simulink model "AariaHIABTorqueR2017a2"  (R2017a)
settings: Solver=VariableStepAuto  StartTime=0.0  StopTime=inf  FixedStep=0.1  RelTol=1e-3  EnableMultiTasking=on
model workspace (MATLAB code in the model file):
  | my_a =1;
undefined symbols (not defined in the file or in its folder): AARIAENV, AARIAMAN, AARIASEN, Camera, sensor, Source_TS, X, Y, Z
libraries: sm_lib x369, nesl_utility x225, dspmathops x92, simulink x70, powerlib_meascontrol x3, vrlib x2, aerolibanimutils x1, aerolibutil x1
(part 9 of 10)

== system AariaHIABTorqueR2017a2/Joint2/RevoluteMotion/IMU Sensors/Sensor Module1/omega_noise ==
  Cumulative Sum : dspmathops/Cumulative Sum  dim=Channels (running sum)  InputProcessing=Columns as channels (frame based)  reset_popup=None  outputDataTypeStr=Inherit: Same as accumulator  outputLastDataTypeStr=Inherit: Same as accumulator  outputMin=[]  outputMax=[]  roundingMode=Floor  overflowMode=off
      settings: SourceProductName=DSP System Toolbox
  Cumulative Sum1 : dspmathops/Cumulative Sum  dim=Channels (running sum)  InputProcessing=Columns as channels (frame based)  reset_popup=None  outputDataTypeStr=Inherit: Same as accumulator  outputLastDataTypeStr=Inherit: Same as accumulator  outputMin=[]  outputMax=[]  roundingMode=Floor  overflowMode=off
      settings: SourceProductName=DSP System Toolbox
  Cumulative Sum2 : dspmathops/Cumulative Sum  dim=Channels (running sum)  InputProcessing=Columns as channels (frame based)  reset_popup=None  outputDataTypeStr=Inherit: Same as accumulator  outputLastDataTypeStr=Inherit: Same as accumulator  outputMin=[]  outputMax=[]  roundingMode=Floor  overflowMode=off
      settings: SourceProductName=DSP System Toolbox
  Gain1 : Gain  Gain=AARIASEN.ErrorGain
  Gain2 : Gain  Gain=AARIASEN.gNormalGain
  Gain3 : Gain  Gain=AARIASEN.gNormalGain
  Gain4 : Gain  Gain=AARIASEN.gNormalGain
  Mux5 : Mux  Inputs=3
  Random Number : RandomNumber  Mean=AARIASEN.gMu  Variance=AARIASEN.gSigma  Seed=AARIASEN.rand(nL,(nS-1)*6+1)  SampleTime=AARIAENV.Source_TS
  Random Number1 : RandomNumber  Mean=AARIASEN.gMu  Variance=AARIASEN.gSigma  Seed=AARIASEN.rand(nL,(nS-1)*6+2)  SampleTime=AARIAENV.Source_TS
  Random Number2 : RandomNumber  Mean=AARIASEN.gMu  Variance=AARIASEN.gSigma  Seed=AARIASEN.rand(nL,(nS-1)*6+3)  SampleTime=AARIAENV.Source_TS
  Sum1 : Sum  Inputs=|++
  Sum2 : Sum  Inputs=|++
  Sum3 : Sum  Inputs=++|
  Sum4 : Sum  Inputs=|++
  gyro in-run bias : simulink/Sources/Ramp  slope=AARIASEN.gBias  start=0  X0=AARIASEN.gInitBias
  gyro random walk : UniformRandomNumber  Minimum=-AARIASEN.gWalk  Maximum=AARIASEN.gWalk  Seed=AARIASEN.rand(nL,(nS-1)*6+1)  SampleTime=AARIAENV.Source_TS
  gyro random walk1 : UniformRandomNumber  Minimum=-AARIASEN.gWalk  Maximum=AARIASEN.gWalk  Seed=AARIASEN.rand(nL,(nS-1)*6+2)  SampleTime=AARIAENV.Source_TS
  gyro random walk2 : UniformRandomNumber  Minimum=-AARIASEN.gWalk  Maximum=AARIASEN.gWalk  Seed=AARIASEN.rand(nL,(nS-1)*6+3)  SampleTime=AARIAENV.Source_TS
  noise : Outport
  wires:
  Gain4/1 -> Sum4/1
  Gain3/1 -> Sum2/1
  Gain2/1 -> Sum1/1
  Random Number/1 -> Gain2/1
  Random Number1/1 -> Gain3/1
  Random Number2/1 -> Gain4/1
  Sum3/1 -> Gain1/1
  Mux5/1 -> Sum3/2
  Sum4/1 -> Mux5/3
  Cumulative Sum2/1 -> Sum4/2
  Cumulative Sum1/1 -> Sum2/2
  Sum2/1 -> Mux5/2
  Sum1/1 -> Mux5/1
  gyro random walk2/1 -> Cumulative Sum2/1
  gyro random walk1/1 -> Cumulative Sum1/1
  Gain1/1 -> noise/1
  gyro random walk/1 -> Cumulative Sum/1
  Cumulative Sum/1 -> Sum1/2
  gyro in-run bias/1 -> Sum3/1

== system AariaHIABTorqueR2017a2/Joint2/RevoluteMotion/IMU Sensors/Sensor Module2/a_noise ==
  Cumulative Sum1 : dspmathops/Cumulative Sum  dim=Channels (running sum)  InputProcessing=Columns as channels (frame based)  reset_popup=None  outputDataTypeStr=Inherit: Same as accumulator  outputLastDataTypeStr=Inherit: Same as accumulator  outputMin=[]  outputMax=[]  roundingMode=Floor  overflowMode=off
      settings: SourceProductName=DSP System Toolbox
  Cumulative Sum2 : dspmathops/Cumulative Sum  dim=Channels (running sum)  InputProcessing=Columns as channels (frame based)  reset_popup=None  outputDataTypeStr=Inherit: Same as accumulator  outputLastDataTypeStr=Inherit: Same as accumulator  outputMin=[]  outputMax=[]  roundingMode=Floor  overflowMode=off
      settings: SourceProductName=DSP System Toolbox
  Cumulative Sum3 : dspmathops/Cumulative Sum  dim=Channels (running sum)  InputProcessing=Columns as channels (frame based)  reset_popup=None  outputDataTypeStr=Inherit: Same as accumulator  outputLastDataTypeStr=Inherit: Same as accumulator  outputMin=[]  outputMax=[]  roundingMode=Floor  overflowMode=off
      settings: SourceProductName=DSP System Toolbox
  Gain1 : Gain  Gain=9.81
  Gain2 : Gain  Gain=AARIASEN.ErrorGain
  Gain3 : Gain  Gain=9.81
  Gain4 : Gain  Gain=AARIASEN.aNormalGain
  Gain5 : Gain  Gain=9.81
  Gain6 : Gain  Gain=AARIASEN.aNormalGain
  Gain7 : Gain  Gain=AARIASEN.aNormalGain
  Mux5 : Mux  Inputs=3
  Random Number : RandomNumber  Mean=AARIASEN.aMu  Variance=AARIASEN.aSigma  Seed=AARIASEN.rand(nL,(nS-1)*6+4)  SampleTime=AARIAENV.Source_TS
  Random Number1 : RandomNumber  Mean=AARIASEN.aMu  Variance=AARIASEN.aSigma  Seed=AARIASEN.rand(nL,(nS-1)*6+5)  SampleTime=AARIAENV.Source_TS
  Random Number2 : RandomNumber  Mean=AARIASEN.aMu  Variance=AARIASEN.aSigma  Seed=AARIASEN.rand(nL,(nS-1)*6+6)  SampleTime=AARIAENV.Source_TS
  Sum1 : Sum  Inputs=|++
  Sum2 : Sum  Inputs=|++
  Sum3 : Sum  Inputs=|++
  Sum4 : Sum  Inputs=++|
  acc in-run bias : simulink/Sources/Ramp  slope=AARIASEN.aBias  start=0  X0=AARIASEN.aInitBias
  acc random walk : UniformRandomNumber  Minimum=-AARIASEN.aWalk  Maximum=AARIASEN.aWalk  Seed=AARIASEN.rand(nL,(nS-1)*6+4)  SampleTime=AARIAENV.Source_TS
  acc random walk1 : UniformRandomNumber  Minimum=-AARIASEN.aWalk  Maximum=AARIASEN.aWalk  Seed=AARIASEN.rand(nL,(nS-1)*6+5)  SampleTime=AARIAENV.Source_TS
  acc random walk2 : UniformRandomNumber  Minimum=-AARIASEN.aWalk  Maximum=AARIASEN.aWalk  Seed=AARIASEN.rand(nL,(nS-1)*6+6)  SampleTime=AARIAENV.Source_TS
  noise : Outport
  wires:
  Gain7/1 -> Gain3/1
  Gain6/1 -> Gain5/1
  Gain4/1 -> Gain1/1
  Random Number2/1 -> Gain7/1
  Random Number1/1 -> Gain6/1
  Random Number/1 -> Gain4/1
  Gain3/1 -> Sum3/1
  Gain5/1 -> Sum2/1
  Gain1/1 -> Sum1/1
  Sum4/1 -> Gain2/1
  Mux5/1 -> Sum4/2
  acc random walk2/1 -> Cumulative Sum3/1
  acc random walk1/1 -> Cumulative Sum1/1
  Sum2/1 -> Mux5/2
  Cumulative Sum1/1 -> Sum2/2
  Sum3/1 -> Mux5/3
  Sum1/1 -> Mux5/1
  Cumulative Sum2/1 -> Sum1/2
  Cumulative Sum3/1 -> Sum3/2
  Gain2/1 -> noise/1
  acc in-run bias/1 -> Sum4/1
  acc random walk/1 -> Cumulative Sum2/1

== system AariaHIABTorqueR2017a2/Joint2/RevoluteMotion/IMU Sensors/Sensor Module2/omega_noise ==
  Cumulative Sum : dspmathops/Cumulative Sum  dim=Channels (running sum)  InputProcessing=Columns as channels (frame based)  reset_popup=None  outputDataTypeStr=Inherit: Same as accumulator  outputLastDataTypeStr=Inherit: Same as accumulator  outputMin=[]  outputMax=[]  roundingMode=Floor  overflowMode=off
      settings: SourceProductName=DSP System Toolbox
  Cumulative Sum1 : dspmathops/Cumulative Sum  dim=Channels (running sum)  InputProcessing=Columns as channels (frame based)  reset_popup=None  outputDataTypeStr=Inherit: Same as accumulator  outputLastDataTypeStr=Inherit: Same as accumulator  outputMin=[]  outputMax=[]  roundingMode=Floor  overflowMode=off
      settings: SourceProductName=DSP System Toolbox
  Cumulative Sum2 : dspmathops/Cumulative Sum  dim=Channels (running sum)  InputProcessing=Columns as channels (frame based)  reset_popup=None  outputDataTypeStr=Inherit: Same as accumulator  outputLastDataTypeStr=Inherit: Same as accumulator  outputMin=[]  outputMax=[]  roundingMode=Floor  overflowMode=off
      settings: SourceProductName=DSP System Toolbox
  Gain1 : Gain  Gain=AARIASEN.ErrorGain
  Gain2 : Gain  Gain=AARIASEN.gNormalGain
  Gain3 : Gain  Gain=AARIASEN.gNormalGain
  Gain4 : Gain  Gain=AARIASEN.gNormalGain
  Mux5 : Mux  Inputs=3
  Random Number : RandomNumber  Mean=AARIASEN.gMu  Variance=AARIASEN.gSigma  Seed=AARIASEN.rand(nL,(nS-1)*6+1)  SampleTime=AARIAENV.Source_TS
  Random Number1 : RandomNumber  Mean=AARIASEN.gMu  Variance=AARIASEN.gSigma  Seed=AARIASEN.rand(nL,(nS-1)*6+2)  SampleTime=AARIAENV.Source_TS
  Random Number2 : RandomNumber  Mean=AARIASEN.gMu  Variance=AARIASEN.gSigma  Seed=AARIASEN.rand(nL,(nS-1)*6+3)  SampleTime=AARIAENV.Source_TS
  Sum1 : Sum  Inputs=|++
  Sum2 : Sum  Inputs=|++
  Sum3 : Sum  Inputs=++|
  Sum4 : Sum  Inputs=|++
  gyro in-run bias : simulink/Sources/Ramp  slope=AARIASEN.gBias  start=0  X0=AARIASEN.gInitBias
  gyro random walk : UniformRandomNumber  Minimum=-AARIASEN.gWalk  Maximum=AARIASEN.gWalk  Seed=AARIASEN.rand(nL,(nS-1)*6+1)  SampleTime=AARIAENV.Source_TS
  gyro random walk1 : UniformRandomNumber  Minimum=-AARIASEN.gWalk  Maximum=AARIASEN.gWalk  Seed=AARIASEN.rand(nL,(nS-1)*6+2)  SampleTime=AARIAENV.Source_TS
  gyro random walk2 : UniformRandomNumber  Minimum=-AARIASEN.gWalk  Maximum=AARIASEN.gWalk  Seed=AARIASEN.rand(nL,(nS-1)*6+3)  SampleTime=AARIAENV.Source_TS
  noise : Outport
  wires:
  Gain4/1 -> Sum4/1
  Gain3/1 -> Sum2/1
  Gain2/1 -> Sum1/1
  Random Number/1 -> Gain2/1
  Random Number1/1 -> Gain3/1
  Random Number2/1 -> Gain4/1
  Sum3/1 -> Gain1/1
  Mux5/1 -> Sum3/2
  Sum4/1 -> Mux5/3
  Cumulative Sum2/1 -> Sum4/2
  Cumulative Sum1/1 -> Sum2/2
  Sum2/1 -> Mux5/2
  Sum1/1 -> Mux5/1
  gyro random walk2/1 -> Cumulative Sum2/1
  gyro random walk1/1 -> Cumulative Sum1/1
  Gain1/1 -> noise/1
  gyro random walk/1 -> Cumulative Sum/1
  Cumulative Sum/1 -> Sum1/2
  gyro in-run bias/1 -> Sum3/1

== system AariaHIABTorqueR2017a2/Joint3/RevoluteMotion/IMU Sensors/Sensor Module1/a_noise ==
  Cumulative Sum1 : dspmathops/Cumulative Sum  dim=Channels (running sum)  InputProcessing=Columns as channels (frame based)  reset_popup=None  outputDataTypeStr=Inherit: Same as accumulator  outputLastDataTypeStr=Inherit: Same as accumulator  outputMin=[]  outputMax=[]  roundingMode=Floor  overflowMode=off
      settings: SourceProductName=DSP System Toolbox
  Cumulative Sum2 : dspmathops/Cumulative Sum  dim=Channels (running sum)  InputProcessing=Columns as channels (frame based)  reset_popup=None  outputDataTypeStr=Inherit: Same as accumulator  outputLastDataTypeStr=Inherit: Same as accumulator  outputMin=[]  outputMax=[]  roundingMode=Floor  overflowMode=off
      settings: SourceProductName=DSP System Toolbox
  Cumulative Sum3 : dspmathops/Cumulative Sum  dim=Channels (running sum)  InputProcessing=Columns as channels (frame based)  reset_popup=None  outputDataTypeStr=Inherit: Same as accumulator  outputLastDataTypeStr=Inherit: Same as accumulator  outputMin=[]  outputMax=[]  roundingMode=Floor  overflowMode=off
      settings: SourceProductName=DSP System Toolbox
  Gain1 : Gain  Gain=9.81
  Gain2 : Gain  Gain=AARIASEN.ErrorGain
  Gain3 : Gain  Gain=9.81
  Gain4 : Gain  Gain=AARIASEN.aNormalGain
  Gain5 : Gain  Gain=9.81
  Gain6 : Gain  Gain=AARIASEN.aNormalGain
  Gain7 : Gain  Gain=AARIASEN.aNormalGain
  Mux5 : Mux  Inputs=3
  Random Number : RandomNumber  Mean=AARIASEN.aMu  Variance=AARIASEN.aSigma  Seed=AARIASEN.rand(nL,(nS-1)*6+4)  SampleTime=AARIAENV.Source_TS
  Random Number1 : RandomNumber  Mean=AARIASEN.aMu  Variance=AARIASEN.aSigma  Seed=AARIASEN.rand(nL,(nS-1)*6+5)  SampleTime=AARIAENV.Source_TS
  Random Number2 : RandomNumber  Mean=AARIASEN.aMu  Variance=AARIASEN.aSigma  Seed=AARIASEN.rand(nL,(nS-1)*6+6)  SampleTime=AARIAENV.Source_TS
  Sum1 : Sum  Inputs=|++
  Sum2 : Sum  Inputs=|++
  Sum3 : Sum  Inputs=|++
  Sum4 : Sum  Inputs=++|
  acc in-run bias : simulink/Sources/Ramp  slope=AARIASEN.aBias  start=0  X0=AARIASEN.aInitBias
  acc random walk : UniformRandomNumber  Minimum=-AARIASEN.aWalk  Maximum=AARIASEN.aWalk  Seed=AARIASEN.rand(nL,(nS-1)*6+4)  SampleTime=AARIAENV.Source_TS
  acc random walk1 : UniformRandomNumber  Minimum=-AARIASEN.aWalk  Maximum=AARIASEN.aWalk  Seed=AARIASEN.rand(nL,(nS-1)*6+5)  SampleTime=AARIAENV.Source_TS
  acc random walk2 : UniformRandomNumber  Minimum=-AARIASEN.aWalk  Maximum=AARIASEN.aWalk  Seed=AARIASEN.rand(nL,(nS-1)*6+6)  SampleTime=AARIAENV.Source_TS
  noise : Outport
  wires:
  Gain7/1 -> Gain3/1
  Gain6/1 -> Gain5/1
  Gain4/1 -> Gain1/1
  Random Number2/1 -> Gain7/1
  Random Number1/1 -> Gain6/1
  Random Number/1 -> Gain4/1
  Gain3/1 -> Sum3/1
  Gain5/1 -> Sum2/1
  Gain1/1 -> Sum1/1
  Sum4/1 -> Gain2/1
  Mux5/1 -> Sum4/2
  acc random walk2/1 -> Cumulative Sum3/1
  acc random walk1/1 -> Cumulative Sum1/1
  Sum2/1 -> Mux5/2
  Cumulative Sum1/1 -> Sum2/2
  Sum3/1 -> Mux5/3
  Sum1/1 -> Mux5/1
  Cumulative Sum2/1 -> Sum1/2
  Cumulative Sum3/1 -> Sum3/2
  Gain2/1 -> noise/1
  acc in-run bias/1 -> Sum4/1
  acc random walk/1 -> Cumulative Sum2/1

== system AariaHIABTorqueR2017a2/Joint3/RevoluteMotion/IMU Sensors/Sensor Module1/omega_noise ==
  Cumulative Sum : dspmathops/Cumulative Sum  dim=Channels (running sum)  InputProcessing=Columns as channels (frame based)  reset_popup=None  outputDataTypeStr=Inherit: Same as accumulator  outputLastDataTypeStr=Inherit: Same as accumulator  outputMin=[]  outputMax=[]  roundingMode=Floor  overflowMode=off
      settings: SourceProductName=DSP System Toolbox
  Cumulative Sum1 : dspmathops/Cumulative Sum  dim=Channels (running sum)  InputProcessing=Columns as channels (frame based)  reset_popup=None  outputDataTypeStr=Inherit: Same as accumulator  outputLastDataTypeStr=Inherit: Same as accumulator  outputMin=[]  outputMax=[]  roundingMode=Floor  overflowMode=off
      settings: SourceProductName=DSP System Toolbox
  Cumulative Sum2 : dspmathops/Cumulative Sum  dim=Channels (running sum)  InputProcessing=Columns as channels (frame based)  reset_popup=None  outputDataTypeStr=Inherit: Same as accumulator  outputLastDataTypeStr=Inherit: Same as accumulator  outputMin=[]  outputMax=[]  roundingMode=Floor  overflowMode=off
      settings: SourceProductName=DSP System Toolbox
  Gain1 : Gain  Gain=AARIASEN.ErrorGain
  Gain2 : Gain  Gain=AARIASEN.gNormalGain
  Gain3 : Gain  Gain=AARIASEN.gNormalGain
  Gain4 : Gain  Gain=AARIASEN.gNormalGain
  Mux5 : Mux  Inputs=3
  Random Number : RandomNumber  Mean=AARIASEN.gMu  Variance=AARIASEN.gSigma  Seed=AARIASEN.rand(nL,(nS-1)*6+1)  SampleTime=AARIAENV.Source_TS
  Random Number1 : RandomNumber  Mean=AARIASEN.gMu  Variance=AARIASEN.gSigma  Seed=AARIASEN.rand(nL,(nS-1)*6+2)  SampleTime=AARIAENV.Source_TS
  Random Number2 : RandomNumber  Mean=AARIASEN.gMu  Variance=AARIASEN.gSigma  Seed=AARIASEN.rand(nL,(nS-1)*6+3)  SampleTime=AARIAENV.Source_TS
  Sum1 : Sum  Inputs=|++
  Sum2 : Sum  Inputs=|++
  Sum3 : Sum  Inputs=++|
  Sum4 : Sum  Inputs=|++
  gyro in-run bias : simulink/Sources/Ramp  slope=AARIASEN.gBias  start=0  X0=AARIASEN.gInitBias
  gyro random walk : UniformRandomNumber  Minimum=-AARIASEN.gWalk  Maximum=AARIASEN.gWalk  Seed=AARIASEN.rand(nL,(nS-1)*6+1)  SampleTime=AARIAENV.Source_TS
  gyro random walk1 : UniformRandomNumber  Minimum=-AARIASEN.gWalk  Maximum=AARIASEN.gWalk  Seed=AARIASEN.rand(nL,(nS-1)*6+2)  SampleTime=AARIAENV.Source_TS
  gyro random walk2 : UniformRandomNumber  Minimum=-AARIASEN.gWalk  Maximum=AARIASEN.gWalk  Seed=AARIASEN.rand(nL,(nS-1)*6+3)  SampleTime=AARIAENV.Source_TS
  noise : Outport
  wires:
  Gain4/1 -> Sum4/1
  Gain3/1 -> Sum2/1
  Gain2/1 -> Sum1/1
  Random Number/1 -> Gain2/1
  Random Number1/1 -> Gain3/1
  Random Number2/1 -> Gain4/1
  Sum3/1 -> Gain1/1
  Mux5/1 -> Sum3/2
  Sum4/1 -> Mux5/3
  Cumulative Sum2/1 -> Sum4/2
  Cumulative Sum1/1 -> Sum2/2
  Sum2/1 -> Mux5/2
  Sum1/1 -> Mux5/1
  gyro random walk2/1 -> Cumulative Sum2/1
  gyro random walk1/1 -> Cumulative Sum1/1
  Gain1/1 -> noise/1
  gyro random walk/1 -> Cumulative Sum/1
  Cumulative Sum/1 -> Sum1/2
  gyro in-run bias/1 -> Sum3/1

== system AariaHIABTorqueR2017a2/Joint3/RevoluteMotion/IMU Sensors/Sensor Module2/a_noise ==
  Cumulative Sum1 : dspmathops/Cumulative Sum  dim=Channels (running sum)  InputProcessing=Columns as channels (frame based)  reset_popup=None  outputDataTypeStr=Inherit: Same as accumulator  outputLastDataTypeStr=Inherit: Same as accumulator  outputMin=[]  outputMax=[]  roundingMode=Floor  overflowMode=off
      settings: SourceProductName=DSP System Toolbox
  Cumulative Sum2 : dspmathops/Cumulative Sum  dim=Channels (running sum)  InputProcessing=Columns as channels (frame based)  reset_popup=None  outputDataTypeStr=Inherit: Same as accumulator  outputLastDataTypeStr=Inherit: Same as accumulator  outputMin=[]  outputMax=[]  roundingMode=Floor  overflowMode=off
      settings: SourceProductName=DSP System Toolbox
  Cumulative Sum3 : dspmathops/Cumulative Sum  dim=Channels (running sum)  InputProcessing=Columns as channels (frame based)  reset_popup=None  outputDataTypeStr=Inherit: Same as accumulator  outputLastDataTypeStr=Inherit: Same as accumulator  outputMin=[]  outputMax=[]  roundingMode=Floor  overflowMode=off
      settings: SourceProductName=DSP System Toolbox
  Gain1 : Gain  Gain=9.81
  Gain2 : Gain  Gain=AARIASEN.ErrorGain
  Gain3 : Gain  Gain=9.81
  Gain4 : Gain  Gain=AARIASEN.aNormalGain
  Gain5 : Gain  Gain=9.81
  Gain6 : Gain  Gain=AARIASEN.aNormalGain
  Gain7 : Gain  Gain=AARIASEN.aNormalGain
  Mux5 : Mux  Inputs=3
  Random Number : RandomNumber  Mean=AARIASEN.aMu  Variance=AARIASEN.aSigma  Seed=AARIASEN.rand(nL,(nS-1)*6+4)  SampleTime=AARIAENV.Source_TS
  Random Number1 : RandomNumber  Mean=AARIASEN.aMu  Variance=AARIASEN.aSigma  Seed=AARIASEN.rand(nL,(nS-1)*6+5)  SampleTime=AARIAENV.Source_TS
  Random Number2 : RandomNumber  Mean=AARIASEN.aMu  Variance=AARIASEN.aSigma  Seed=AARIASEN.rand(nL,(nS-1)*6+6)  SampleTime=AARIAENV.Source_TS
  Sum1 : Sum  Inputs=|++
  Sum2 : Sum  Inputs=|++
  Sum3 : Sum  Inputs=|++
  Sum4 : Sum  Inputs=++|
  acc in-run bias : simulink/Sources/Ramp  slope=AARIASEN.aBias  start=0  X0=AARIASEN.aInitBias
  acc random walk : UniformRandomNumber  Minimum=-AARIASEN.aWalk  Maximum=AARIASEN.aWalk  Seed=AARIASEN.rand(nL,(nS-1)*6+4)  SampleTime=AARIAENV.Source_TS
  acc random walk1 : UniformRandomNumber  Minimum=-AARIASEN.aWalk  Maximum=AARIASEN.aWalk  Seed=AARIASEN.rand(nL,(nS-1)*6+5)  SampleTime=AARIAENV.Source_TS
  acc random walk2 : UniformRandomNumber  Minimum=-AARIASEN.aWalk  Maximum=AARIASEN.aWalk  Seed=AARIASEN.rand(nL,(nS-1)*6+6)  SampleTime=AARIAENV.Source_TS
  noise : Outport
  wires:
  Gain7/1 -> Gain3/1
  Gain6/1 -> Gain5/1
  Gain4/1 -> Gain1/1
  Random Number2/1 -> Gain7/1
  Random Number1/1 -> Gain6/1
  Random Number/1 -> Gain4/1
  Gain3/1 -> Sum3/1
  Gain5/1 -> Sum2/1
  Gain1/1 -> Sum1/1
  Sum4/1 -> Gain2/1
  Mux5/1 -> Sum4/2
  acc random walk2/1 -> Cumulative Sum3/1
  acc random walk1/1 -> Cumulative Sum1/1
  Sum2/1 -> Mux5/2
  Cumulative Sum1/1 -> Sum2/2
  Sum3/1 -> Mux5/3
  Sum1/1 -> Mux5/1
  Cumulative Sum2/1 -> Sum1/2
  Cumulative Sum3/1 -> Sum3/2
  Gain2/1 -> noise/1
  acc in-run bias/1 -> Sum4/1
  acc random walk/1 -> Cumulative Sum2/1

== system AariaHIABTorqueR2017a2/Joint3/RevoluteMotion/IMU Sensors/Sensor Module2/omega_noise ==
  Cumulative Sum : dspmathops/Cumulative Sum  dim=Channels (running sum)  InputProcessing=Columns as channels (frame based)  reset_popup=None  outputDataTypeStr=Inherit: Same as accumulator  outputLastDataTypeStr=Inherit: Same as accumulator  outputMin=[]  outputMax=[]  roundingMode=Floor  overflowMode=off
      settings: SourceProductName=DSP System Toolbox
  Cumulative Sum1 : dspmathops/Cumulative Sum  dim=Channels (running sum)  InputProcessing=Columns as channels (frame based)  reset_popup=None  outputDataTypeStr=Inherit: Same as accumulator  outputLastDataTypeStr=Inherit: Same as accumulator  outputMin=[]  outputMax=[]  roundingMode=Floor  overflowMode=off
      settings: SourceProductName=DSP System Toolbox
  Cumulative Sum2 : dspmathops/Cumulative Sum  dim=Channels (running sum)  InputProcessing=Columns as channels (frame based)  reset_popup=None  outputDataTypeStr=Inherit: Same as accumulator  outputLastDataTypeStr=Inherit: Same as accumulator  outputMin=[]  outputMax=[]  roundingMode=Floor  overflowMode=off
      settings: SourceProductName=DSP System Toolbox
  Gain1 : Gain  Gain=AARIASEN.ErrorGain
  Gain2 : Gain  Gain=AARIASEN.gNormalGain
  Gain3 : Gain  Gain=AARIASEN.gNormalGain
  Gain4 : Gain  Gain=AARIASEN.gNormalGain
  Mux5 : Mux  Inputs=3
  Random Number : RandomNumber  Mean=AARIASEN.gMu  Variance=AARIASEN.gSigma  Seed=AARIASEN.rand(nL,(nS-1)*6+1)  SampleTime=AARIAENV.Source_TS
  Random Number1 : RandomNumber  Mean=AARIASEN.gMu  Variance=AARIASEN.gSigma  Seed=AARIASEN.rand(nL,(nS-1)*6+2)  SampleTime=AARIAENV.Source_TS
  Random Number2 : RandomNumber  Mean=AARIASEN.gMu  Variance=AARIASEN.gSigma  Seed=AARIASEN.rand(nL,(nS-1)*6+3)  SampleTime=AARIAENV.Source_TS
  Sum1 : Sum  Inputs=|++
  Sum2 : Sum  Inputs=|++
  Sum3 : Sum  Inputs=++|
  Sum4 : Sum  Inputs=|++
  gyro in-run bias : simulink/Sources/Ramp  slope=AARIASEN.gBias  start=0  X0=AARIASEN.gInitBias
  gyro random walk : UniformRandomNumber  Minimum=-AARIASEN.gWalk  Maximum=AARIASEN.gWalk  Seed=AARIASEN.rand(nL,(nS-1)*6+1)  SampleTime=AARIAENV.Source_TS
  gyro random walk1 : UniformRandomNumber  Minimum=-AARIASEN.gWalk  Maximum=AARIASEN.gWalk  Seed=AARIASEN.rand(nL,(nS-1)*6+2)  SampleTime=AARIAENV.Source_TS
  gyro random walk2 : UniformRandomNumber  Minimum=-AARIASEN.gWalk  Maximum=AARIASEN.gWalk  Seed=AARIASEN.rand(nL,(nS-1)*6+3)  SampleTime=AARIAENV.Source_TS
  noise : Outport
  wires:
  Gain4/1 -> Sum4/1
  Gain3/1 -> Sum2/1
  Gain2/1 -> Sum1/1
  Random Number/1 -> Gain2/1
  Random Number1/1 -> Gain3/1
  Random Number2/1 -> Gain4/1
  Sum3/1 -> Gain1/1
  Mux5/1 -> Sum3/2
  Sum4/1 -> Mux5/3
  Cumulative Sum2/1 -> Sum4/2
  Cumulative Sum1/1 -> Sum2/2
  Sum2/1 -> Mux5/2
  Sum1/1 -> Mux5/1
  gyro random walk2/1 -> Cumulative Sum2/1
  gyro random walk1/1 -> Cumulative Sum1/1
  Gain1/1 -> noise/1
  gyro random walk/1 -> Cumulative Sum/1
  Cumulative Sum/1 -> Sum1/2
  gyro in-run bias/1 -> Sum3/1

== system AariaHIABTorqueR2017a2/Joint4/PrismaticMotion/IMU Sensors/Sensor Module1/a_noise ==
  Cumulative Sum1 : dspmathops/Cumulative Sum  dim=Channels (running sum)  InputProcessing=Columns as channels (frame based)  reset_popup=None  outputDataTypeStr=Inherit: Same as accumulator  outputLastDataTypeStr=Inherit: Same as accumulator  outputMin=[]  outputMax=[]  roundingMode=Floor  overflowMode=off
      settings: SourceProductName=DSP System Toolbox
  Cumulative Sum2 : dspmathops/Cumulative Sum  dim=Channels (running sum)  InputProcessing=Columns as channels (frame based)  reset_popup=None  outputDataTypeStr=Inherit: Same as accumulator  outputLastDataTypeStr=Inherit: Same as accumulator  outputMin=[]  outputMax=[]  roundingMode=Floor  overflowMode=off
      settings: SourceProductName=DSP System Toolbox
  Cumulative Sum3 : dspmathops/Cumulative Sum  dim=Channels (running sum)  InputProcessing=Columns as channels (frame based)  reset_popup=None  outputDataTypeStr=Inherit: Same as accumulator  outputLastDataTypeStr=Inherit: Same as accumulator  outputMin=[]  outputMax=[]  roundingMode=Floor  overflowMode=off
      settings: SourceProductName=DSP System Toolbox
  Gain1 : Gain  Gain=9.81
  Gain2 : Gain  Gain=AARIASEN.ErrorGain
  Gain3 : Gain  Gain=9.81
  Gain4 : Gain  Gain=AARIASEN.aNormalGain
  Gain5 : Gain  Gain=9.81
  Gain6 : Gain  Gain=AARIASEN.aNormalGain
  Gain7 : Gain  Gain=AARIASEN.aNormalGain
  Mux5 : Mux  Inputs=3
  Random Number : RandomNumber  Mean=AARIASEN.aMu  Variance=AARIASEN.aSigma  Seed=AARIASEN.rand(nL,(nS-1)*6+4)  SampleTime=AARIAENV.Source_TS
  Random Number1 : RandomNumber  Mean=AARIASEN.aMu  Variance=AARIASEN.aSigma  Seed=AARIASEN.rand(nL,(nS-1)*6+5)  SampleTime=AARIAENV.Source_TS
  Random Number2 : RandomNumber  Mean=AARIASEN.aMu  Variance=AARIASEN.aSigma  Seed=AARIASEN.rand(nL,(nS-1)*6+6)  SampleTime=AARIAENV.Source_TS
  Sum1 : Sum  Inputs=|++
  Sum2 : Sum  Inputs=|++
  Sum3 : Sum  Inputs=|++
  Sum4 : Sum  Inputs=++|
  acc in-run bias : simulink/Sources/Ramp  slope=AARIASEN.aBias  start=0  X0=AARIASEN.aInitBias
  acc random walk : UniformRandomNumber  Minimum=-AARIASEN.aWalk  Maximum=AARIASEN.aWalk  Seed=AARIASEN.rand(nL,(nS-1)*6+4)  SampleTime=AARIAENV.Source_TS
  acc random walk1 : UniformRandomNumber  Minimum=-AARIASEN.aWalk  Maximum=AARIASEN.aWalk  Seed=AARIASEN.rand(nL,(nS-1)*6+5)  SampleTime=AARIAENV.Source_TS
  acc random walk2 : UniformRandomNumber  Minimum=-AARIASEN.aWalk  Maximum=AARIASEN.aWalk  Seed=AARIASEN.rand(nL,(nS-1)*6+6)  SampleTime=AARIAENV.Source_TS
  noise : Outport
  wires:
  acc random walk/1 -> Cumulative Sum2/1
  acc in-run bias/1 -> Sum4/1
  Gain2/1 -> noise/1
  Cumulative Sum3/1 -> Sum3/2
  Cumulative Sum2/1 -> Sum1/2
  Sum1/1 -> Mux5/1
  Sum3/1 -> Mux5/3
  Cumulative Sum1/1 -> Sum2/2
  Sum2/1 -> Mux5/2
  acc random walk1/1 -> Cumulative Sum1/1
  acc random walk2/1 -> Cumulative Sum3/1
  Mux5/1 -> Sum4/2
  Sum4/1 -> Gain2/1
  Gain1/1 -> Sum1/1
  Gain5/1 -> Sum2/1
  Gain3/1 -> Sum3/1
  Random Number/1 -> Gain4/1
  Random Number1/1 -> Gain6/1
  Random Number2/1 -> Gain7/1
  Gain4/1 -> Gain1/1
  Gain6/1 -> Gain5/1
  Gain7/1 -> Gain3/1

== system AariaHIABTorqueR2017a2/Joint4/PrismaticMotion/IMU Sensors/Sensor Module1/omega_noise ==
  Cumulative Sum : dspmathops/Cumulative Sum  dim=Channels (running sum)  InputProcessing=Columns as channels (frame based)  reset_popup=None  outputDataTypeStr=Inherit: Same as accumulator  outputLastDataTypeStr=Inherit: Same as accumulator  outputMin=[]  outputMax=[]  roundingMode=Floor  overflowMode=off
      settings: SourceProductName=DSP System Toolbox
  Cumulative Sum1 : dspmathops/Cumulative Sum  dim=Channels (running sum)  InputProcessing=Columns as channels (frame based)  reset_popup=None  outputDataTypeStr=Inherit: Same as accumulator  outputLastDataTypeStr=Inherit: Same as accumulator  outputMin=[]  outputMax=[]  roundingMode=Floor  overflowMode=off
      settings: SourceProductName=DSP System Toolbox
  Cumulative Sum2 : dspmathops/Cumulative Sum  dim=Channels (running sum)  InputProcessing=Columns as channels (frame based)  reset_popup=None  outputDataTypeStr=Inherit: Same as accumulator  outputLastDataTypeStr=Inherit: Same as accumulator  outputMin=[]  outputMax=[]  roundingMode=Floor  overflowMode=off
      settings: SourceProductName=DSP System Toolbox
  Gain1 : Gain  Gain=AARIASEN.ErrorGain
  Gain2 : Gain  Gain=AARIASEN.gNormalGain
  Gain3 : Gain  Gain=AARIASEN.gNormalGain
  Gain4 : Gain  Gain=AARIASEN.gNormalGain
  Mux5 : Mux  Inputs=3
  Random Number : RandomNumber  Mean=AARIASEN.gMu  Variance=AARIASEN.gSigma  Seed=AARIASEN.rand(nL,(nS-1)*6+1)  SampleTime=AARIAENV.Source_TS
  Random Number1 : RandomNumber  Mean=AARIASEN.gMu  Variance=AARIASEN.gSigma  Seed=AARIASEN.rand(nL,(nS-1)*6+2)  SampleTime=AARIAENV.Source_TS
  Random Number2 : RandomNumber  Mean=AARIASEN.gMu  Variance=AARIASEN.gSigma  Seed=AARIASEN.rand(nL,(nS-1)*6+3)  SampleTime=AARIAENV.Source_TS
  Sum1 : Sum  Inputs=|++
  Sum2 : Sum  Inputs=|++
  Sum3 : Sum  Inputs=++|
  Sum4 : Sum  Inputs=|++
  gyro in-run bias : simulink/Sources/Ramp  slope=AARIASEN.gBias  start=0  X0=AARIASEN.gInitBias
  gyro random walk : UniformRandomNumber  Minimum=-AARIASEN.gWalk  Maximum=AARIASEN.gWalk  Seed=AARIASEN.rand(nL,(nS-1)*6+1)  SampleTime=AARIAENV.Source_TS
  gyro random walk1 : UniformRandomNumber  Minimum=-AARIASEN.gWalk  Maximum=AARIASEN.gWalk  Seed=AARIASEN.rand(nL,(nS-1)*6+2)  SampleTime=AARIAENV.Source_TS
  gyro random walk2 : UniformRandomNumber  Minimum=-AARIASEN.gWalk  Maximum=AARIASEN.gWalk  Seed=AARIASEN.rand(nL,(nS-1)*6+3)  SampleTime=AARIAENV.Source_TS
  noise : Outport
  wires:
  gyro in-run bias/1 -> Sum3/1
  Cumulative Sum/1 -> Sum1/2
  gyro random walk/1 -> Cumulative Sum/1
  Gain1/1 -> noise/1
  gyro random walk1/1 -> Cumulative Sum1/1
  gyro random walk2/1 -> Cumulative Sum2/1
  Sum1/1 -> Mux5/1
  Sum2/1 -> Mux5/2
  Cumulative Sum1/1 -> Sum2/2
  Cumulative Sum2/1 -> Sum4/2
  Sum4/1 -> Mux5/3
  Mux5/1 -> Sum3/2
  Sum3/1 -> Gain1/1
  Random Number2/1 -> Gain4/1
  Random Number1/1 -> Gain3/1
  Random Number/1 -> Gain2/1
  Gain2/1 -> Sum1/1
  Gain3/1 -> Sum2/1
  Gain4/1 -> Sum4/1

== system AariaHIABTorqueR2017a2/Joint4/PrismaticMotion/IMU Sensors/Sensor Module2/a_noise ==
  Cumulative Sum1 : dspmathops/Cumulative Sum  dim=Channels (running sum)  InputProcessing=Columns as channels (frame based)  reset_popup=None  outputDataTypeStr=Inherit: Same as accumulator  outputLastDataTypeStr=Inherit: Same as accumulator  outputMin=[]  outputMax=[]  roundingMode=Floor  overflowMode=off
      settings: SourceProductName=DSP System Toolbox
  Cumulative Sum2 : dspmathops/Cumulative Sum  dim=Channels (running sum)  InputProcessing=Columns as channels (frame based)  reset_popup=None  outputDataTypeStr=Inherit: Same as accumulator  outputLastDataTypeStr=Inherit: Same as accumulator  outputMin=[]  outputMax=[]  roundingMode=Floor  overflowMode=off
      settings: SourceProductName=DSP System Toolbox
  Cumulative Sum3 : dspmathops/Cumulative Sum  dim=Channels (running sum)  InputProcessing=Columns as channels (frame based)  reset_popup=None  outputDataTypeStr=Inherit: Same as accumulator  outputLastDataTypeStr=Inherit: Same as accumulator  outputMin=[]  outputMax=[]  roundingMode=Floor  overflowMode=off
      settings: SourceProductName=DSP System Toolbox
  Gain1 : Gain  Gain=9.81
  Gain2 : Gain  Gain=AARIASEN.ErrorGain
  Gain3 : Gain  Gain=9.81
  Gain4 : Gain  Gain=AARIASEN.aNormalGain
  Gain5 : Gain  Gain=9.81
  Gain6 : Gain  Gain=AARIASEN.aNormalGain
  Gain7 : Gain  Gain=AARIASEN.aNormalGain
  Mux5 : Mux  Inputs=3
  Random Number : RandomNumber  Mean=AARIASEN.aMu  Variance=AARIASEN.aSigma  Seed=AARIASEN.rand(nL,(nS-1)*6+4)  SampleTime=AARIAENV.Source_TS
  Random Number1 : RandomNumber  Mean=AARIASEN.aMu  Variance=AARIASEN.aSigma  Seed=AARIASEN.rand(nL,(nS-1)*6+5)  SampleTime=AARIAENV.Source_TS
  Random Number2 : RandomNumber  Mean=AARIASEN.aMu  Variance=AARIASEN.aSigma  Seed=AARIASEN.rand(nL,(nS-1)*6+6)  SampleTime=AARIAENV.Source_TS
  Sum1 : Sum  Inputs=|++
  Sum2 : Sum  Inputs=|++
  Sum3 : Sum  Inputs=|++
  Sum4 : Sum  Inputs=++|
  acc in-run bias : simulink/Sources/Ramp  slope=AARIASEN.aBias  start=0  X0=AARIASEN.aInitBias
  acc random walk : UniformRandomNumber  Minimum=-AARIASEN.aWalk  Maximum=AARIASEN.aWalk  Seed=AARIASEN.rand(nL,(nS-1)*6+4)  SampleTime=AARIAENV.Source_TS
  acc random walk1 : UniformRandomNumber  Minimum=-AARIASEN.aWalk  Maximum=AARIASEN.aWalk  Seed=AARIASEN.rand(nL,(nS-1)*6+5)  SampleTime=AARIAENV.Source_TS
  acc random walk2 : UniformRandomNumber  Minimum=-AARIASEN.aWalk  Maximum=AARIASEN.aWalk  Seed=AARIASEN.rand(nL,(nS-1)*6+6)  SampleTime=AARIAENV.Source_TS
  noise : Outport
  wires:
  acc random walk/1 -> Cumulative Sum2/1
  acc in-run bias/1 -> Sum4/1
  Gain2/1 -> noise/1
  Cumulative Sum3/1 -> Sum3/2
  Cumulative Sum2/1 -> Sum1/2
  Sum1/1 -> Mux5/1
  Sum3/1 -> Mux5/3
  Cumulative Sum1/1 -> Sum2/2
  Sum2/1 -> Mux5/2
  acc random walk1/1 -> Cumulative Sum1/1
  acc random walk2/1 -> Cumulative Sum3/1
  Mux5/1 -> Sum4/2
  Sum4/1 -> Gain2/1
  Gain1/1 -> Sum1/1
  Gain5/1 -> Sum2/1
  Gain3/1 -> Sum3/1
  Random Number/1 -> Gain4/1
  Random Number1/1 -> Gain6/1
  Random Number2/1 -> Gain7/1
  Gain4/1 -> Gain1/1
  Gain6/1 -> Gain5/1
  Gain7/1 -> Gain3/1

== system AariaHIABTorqueR2017a2/Joint4/PrismaticMotion/IMU Sensors/Sensor Module2/omega_noise ==
  Cumulative Sum : dspmathops/Cumulative Sum  dim=Channels (running sum)  InputProcessing=Columns as channels (frame based)  reset_popup=None  outputDataTypeStr=Inherit: Same as accumulator  outputLastDataTypeStr=Inherit: Same as accumulator  outputMin=[]  outputMax=[]  roundingMode=Floor  overflowMode=off
      settings: SourceProductName=DSP System Toolbox
  Cumulative Sum1 : dspmathops/Cumulative Sum  dim=Channels (running sum)  InputProcessing=Columns as channels (frame based)  reset_popup=None  outputDataTypeStr=Inherit: Same as accumulator  outputLastDataTypeStr=Inherit: Same as accumulator  outputMin=[]  outputMax=[]  roundingMode=Floor  overflowMode=off
      settings: SourceProductName=DSP System Toolbox
  Cumulative Sum2 : dspmathops/Cumulative Sum  dim=Channels (running sum)  InputProcessing=Columns as channels (frame based)  reset_popup=None  outputDataTypeStr=Inherit: Same as accumulator  outputLastDataTypeStr=Inherit: Same as accumulator  outputMin=[]  outputMax=[]  roundingMode=Floor  overflowMode=off
      settings: SourceProductName=DSP System Toolbox
  Gain1 : Gain  Gain=AARIASEN.ErrorGain
  Gain2 : Gain  Gain=AARIASEN.gNormalGain
  Gain3 : Gain  Gain=AARIASEN.gNormalGain
  Gain4 : Gain  Gain=AARIASEN.gNormalGain
  Mux5 : Mux  Inputs=3
  Random Number : RandomNumber  Mean=AARIASEN.gMu  Variance=AARIASEN.gSigma  Seed=AARIASEN.rand(nL,(nS-1)*6+1)  SampleTime=AARIAENV.Source_TS
  Random Number1 : RandomNumber  Mean=AARIASEN.gMu  Variance=AARIASEN.gSigma  Seed=AARIASEN.rand(nL,(nS-1)*6+2)  SampleTime=AARIAENV.Source_TS
  Random Number2 : RandomNumber  Mean=AARIASEN.gMu  Variance=AARIASEN.gSigma  Seed=AARIASEN.rand(nL,(nS-1)*6+3)  SampleTime=AARIAENV.Source_TS
  Sum1 : Sum  Inputs=|++
  Sum2 : Sum  Inputs=|++
  Sum3 : Sum  Inputs=++|
  Sum4 : Sum  Inputs=|++
  gyro in-run bias : simulink/Sources/Ramp  slope=AARIASEN.gBias  start=0  X0=AARIASEN.gInitBias
  gyro random walk : UniformRandomNumber  Minimum=-AARIASEN.gWalk  Maximum=AARIASEN.gWalk  Seed=AARIASEN.rand(nL,(nS-1)*6+1)  SampleTime=AARIAENV.Source_TS
  gyro random walk1 : UniformRandomNumber  Minimum=-AARIASEN.gWalk  Maximum=AARIASEN.gWalk  Seed=AARIASEN.rand(nL,(nS-1)*6+2)  SampleTime=AARIAENV.Source_TS
  gyro random walk2 : UniformRandomNumber  Minimum=-AARIASEN.gWalk  Maximum=AARIASEN.gWalk  Seed=AARIASEN.rand(nL,(nS-1)*6+3)  SampleTime=AARIAENV.Source_TS
  noise : Outport
  wires:
  gyro in-run bias/1 -> Sum3/1
  Cumulative Sum/1 -> Sum1/2
  gyro random walk/1 -> Cumulative Sum/1
  Gain1/1 -> noise/1
  gyro random walk1/1 -> Cumulative Sum1/1
  gyro random walk2/1 -> Cumulative Sum2/1
  Sum1/1 -> Mux5/1
  Sum2/1 -> Mux5/2
  Cumulative Sum1/1 -> Sum2/2
  Cumulative Sum2/1 -> Sum4/2
  Sum4/1 -> Mux5/3
  Mux5/1 -> Sum3/2
  Sum3/1 -> Gain1/1
  Random Number2/1 -> Gain4/1
  Random Number1/1 -> Gain3/1
  Random Number/1 -> Gain2/1
  Gain2/1 -> Sum1/1
  Gain3/1 -> Sum2/1
  Gain4/1 -> Sum4/1

== system AariaHIABTorqueR2017a2/Joint5/RevoluteMotion/IMU Sensors/Sensor Module1/a_noise ==
  Cumulative Sum1 : dspmathops/Cumulative Sum  dim=Channels (running sum)  InputProcessing=Columns as channels (frame based)  reset_popup=None  outputDataTypeStr=Inherit: Same as accumulator  outputLastDataTypeStr=Inherit: Same as accumulator  outputMin=[]  outputMax=[]  roundingMode=Floor  overflowMode=off
      settings: SourceProductName=DSP System Toolbox
  Cumulative Sum2 : dspmathops/Cumulative Sum  dim=Channels (running sum)  InputProcessing=Columns as channels (frame based)  reset_popup=None  outputDataTypeStr=Inherit: Same as accumulator  outputLastDataTypeStr=Inherit: Same as accumulator  outputMin=[]  outputMax=[]  roundingMode=Floor  overflowMode=off
      settings: SourceProductName=DSP System Toolbox
  Cumulative Sum3 : dspmathops/Cumulative Sum  dim=Channels (running sum)  InputProcessing=Columns as channels (frame based)  reset_popup=None  outputDataTypeStr=Inherit: Same as accumulator  outputLastDataTypeStr=Inherit: Same as accumulator  outputMin=[]  outputMax=[]  roundingMode=Floor  overflowMode=off
      settings: SourceProductName=DSP System Toolbox
  Gain1 : Gain  Gain=9.81
  Gain2 : Gain  Gain=AARIASEN.ErrorGain
  Gain3 : Gain  Gain=9.81
  Gain4 : Gain  Gain=AARIASEN.aNormalGain
  Gain5 : Gain  Gain=9.81
  Gain6 : Gain  Gain=AARIASEN.aNormalGain
  Gain7 : Gain  Gain=AARIASEN.aNormalGain
  Mux5 : Mux  Inputs=3
  Random Number : RandomNumber  Mean=AARIASEN.aMu  Variance=AARIASEN.aSigma  Seed=AARIASEN.rand(nL,(nS-1)*6+4)  SampleTime=AARIAENV.Source_TS
  Random Number1 : RandomNumber  Mean=AARIASEN.aMu  Variance=AARIASEN.aSigma  Seed=AARIASEN.rand(nL,(nS-1)*6+5)  SampleTime=AARIAENV.Source_TS
  Random Number2 : RandomNumber  Mean=AARIASEN.aMu  Variance=AARIASEN.aSigma  Seed=AARIASEN.rand(nL,(nS-1)*6+6)  SampleTime=AARIAENV.Source_TS
  Sum1 : Sum  Inputs=|++
  Sum2 : Sum  Inputs=|++
  Sum3 : Sum  Inputs=|++
  Sum4 : Sum  Inputs=++|
  acc in-run bias : simulink/Sources/Ramp  slope=AARIASEN.aBias  start=0  X0=AARIASEN.aInitBias
  acc random walk : UniformRandomNumber  Minimum=-AARIASEN.aWalk  Maximum=AARIASEN.aWalk  Seed=AARIASEN.rand(nL,(nS-1)*6+4)  SampleTime=AARIAENV.Source_TS
  acc random walk1 : UniformRandomNumber  Minimum=-AARIASEN.aWalk  Maximum=AARIASEN.aWalk  Seed=AARIASEN.rand(nL,(nS-1)*6+5)  SampleTime=AARIAENV.Source_TS
  acc random walk2 : UniformRandomNumber  Minimum=-AARIASEN.aWalk  Maximum=AARIASEN.aWalk  Seed=AARIASEN.rand(nL,(nS-1)*6+6)  SampleTime=AARIAENV.Source_TS
  noise : Outport
  wires:
  acc random walk/1 -> Cumulative Sum2/1
  acc in-run bias/1 -> Sum4/1
  Gain2/1 -> noise/1
  Cumulative Sum3/1 -> Sum3/2
  Cumulative Sum2/1 -> Sum1/2
  Sum1/1 -> Mux5/1
  Sum3/1 -> Mux5/3
  Cumulative Sum1/1 -> Sum2/2
  Sum2/1 -> Mux5/2
  acc random walk1/1 -> Cumulative Sum1/1
  acc random walk2/1 -> Cumulative Sum3/1
  Mux5/1 -> Sum4/2
  Sum4/1 -> Gain2/1
  Gain1/1 -> Sum1/1
  Gain5/1 -> Sum2/1
  Gain3/1 -> Sum3/1
  Random Number/1 -> Gain4/1
  Random Number1/1 -> Gain6/1
  Random Number2/1 -> Gain7/1
  Gain4/1 -> Gain1/1
  Gain6/1 -> Gain5/1
  Gain7/1 -> Gain3/1

== system AariaHIABTorqueR2017a2/Joint5/RevoluteMotion/IMU Sensors/Sensor Module1/omega_noise ==
  Cumulative Sum : dspmathops/Cumulative Sum  dim=Channels (running sum)  InputProcessing=Columns as channels (frame based)  reset_popup=None  outputDataTypeStr=Inherit: Same as accumulator  outputLastDataTypeStr=Inherit: Same as accumulator  outputMin=[]  outputMax=[]  roundingMode=Floor  overflowMode=off
      settings: SourceProductName=DSP System Toolbox
  Cumulative Sum1 : dspmathops/Cumulative Sum  dim=Channels (running sum)  InputProcessing=Columns as channels (frame based)  reset_popup=None  outputDataTypeStr=Inherit: Same as accumulator  outputLastDataTypeStr=Inherit: Same as accumulator  outputMin=[]  outputMax=[]  roundingMode=Floor  overflowMode=off
      settings: SourceProductName=DSP System Toolbox
  Cumulative Sum2 : dspmathops/Cumulative Sum  dim=Channels (running sum)  InputProcessing=Columns as channels (frame based)  reset_popup=None  outputDataTypeStr=Inherit: Same as accumulator  outputLastDataTypeStr=Inherit: Same as accumulator  outputMin=[]  outputMax=[]  roundingMode=Floor  overflowMode=off
      settings: SourceProductName=DSP System Toolbox
  Gain1 : Gain  Gain=AARIASEN.ErrorGain
  Gain2 : Gain  Gain=AARIASEN.gNormalGain
  Gain3 : Gain  Gain=AARIASEN.gNormalGain
  Gain4 : Gain  Gain=AARIASEN.gNormalGain
  Mux5 : Mux  Inputs=3
  Random Number : RandomNumber  Mean=AARIASEN.gMu  Variance=AARIASEN.gSigma  Seed=AARIASEN.rand(nL,(nS-1)*6+1)  SampleTime=AARIAENV.Source_TS
  Random Number1 : RandomNumber  Mean=AARIASEN.gMu  Variance=AARIASEN.gSigma  Seed=AARIASEN.rand(nL,(nS-1)*6+2)  SampleTime=AARIAENV.Source_TS
  Random Number2 : RandomNumber  Mean=AARIASEN.gMu  Variance=AARIASEN.gSigma  Seed=AARIASEN.rand(nL,(nS-1)*6+3)  SampleTime=AARIAENV.Source_TS
  Sum1 : Sum  Inputs=|++
  Sum2 : Sum  Inputs=|++
  Sum3 : Sum  Inputs=++|
  Sum4 : Sum  Inputs=|++
  gyro in-run bias : simulink/Sources/Ramp  slope=AARIASEN.gBias  start=0  X0=AARIASEN.gInitBias
  gyro random walk : UniformRandomNumber  Minimum=-AARIASEN.gWalk  Maximum=AARIASEN.gWalk  Seed=AARIASEN.rand(nL,(nS-1)*6+1)  SampleTime=AARIAENV.Source_TS
  gyro random walk1 : UniformRandomNumber  Minimum=-AARIASEN.gWalk  Maximum=AARIASEN.gWalk  Seed=AARIASEN.rand(nL,(nS-1)*6+2)  SampleTime=AARIAENV.Source_TS
  gyro random walk2 : UniformRandomNumber  Minimum=-AARIASEN.gWalk  Maximum=AARIASEN.gWalk  Seed=AARIASEN.rand(nL,(nS-1)*6+3)  SampleTime=AARIAENV.Source_TS
  noise : Outport
  wires:
  gyro in-run bias/1 -> Sum3/1
  Cumulative Sum/1 -> Sum1/2
  gyro random walk/1 -> Cumulative Sum/1
  Gain1/1 -> noise/1
  gyro random walk1/1 -> Cumulative Sum1/1
  gyro random walk2/1 -> Cumulative Sum2/1
  Sum1/1 -> Mux5/1
  Sum2/1 -> Mux5/2
  Cumulative Sum1/1 -> Sum2/2
  Cumulative Sum2/1 -> Sum4/2
  Sum4/1 -> Mux5/3
  Mux5/1 -> Sum3/2
  Sum3/1 -> Gain1/1
  Random Number2/1 -> Gain4/1
  Random Number1/1 -> Gain3/1
  Random Number/1 -> Gain2/1
  Gain2/1 -> Sum1/1
  Gain3/1 -> Sum2/1
  Gain4/1 -> Sum4/1

== system AariaHIABTorqueR2017a2/Joint5/RevoluteMotion/IMU Sensors/Sensor Module2/a_noise ==
  Cumulative Sum1 : dspmathops/Cumulative Sum  dim=Channels (running sum)  InputProcessing=Columns as channels (frame based)  reset_popup=None  outputDataTypeStr=Inherit: Same as accumulator  outputLastDataTypeStr=Inherit: Same as accumulator  outputMin=[]  outputMax=[]  roundingMode=Floor  overflowMode=off
      settings: SourceProductName=DSP System Toolbox
  Cumulative Sum2 : dspmathops/Cumulative Sum  dim=Channels (running sum)  InputProcessing=Columns as channels (frame based)  reset_popup=None  outputDataTypeStr=Inherit: Same as accumulator  outputLastDataTypeStr=Inherit: Same as accumulator  outputMin=[]  outputMax=[]  roundingMode=Floor  overflowMode=off
      settings: SourceProductName=DSP System Toolbox
  Cumulative Sum3 : dspmathops/Cumulative Sum  dim=Channels (running sum)  InputProcessing=Columns as channels (frame based)  reset_popup=None  outputDataTypeStr=Inherit: Same as accumulator  outputLastDataTypeStr=Inherit: Same as accumulator  outputMin=[]  outputMax=[]  roundingMode=Floor  overflowMode=off
      settings: SourceProductName=DSP System Toolbox
  Gain1 : Gain  Gain=9.81
  Gain2 : Gain  Gain=AARIASEN.ErrorGain
  Gain3 : Gain  Gain=9.81
  Gain4 : Gain  Gain=AARIASEN.aNormalGain
  Gain5 : Gain  Gain=9.81
  Gain6 : Gain  Gain=AARIASEN.aNormalGain
  Gain7 : Gain  Gain=AARIASEN.aNormalGain
  Mux5 : Mux  Inputs=3
  Random Number : RandomNumber  Mean=AARIASEN.aMu  Variance=AARIASEN.aSigma  Seed=AARIASEN.rand(nL,(nS-1)*6+4)  SampleTime=AARIAENV.Source_TS
  Random Number1 : RandomNumber  Mean=AARIASEN.aMu  Variance=AARIASEN.aSigma  Seed=AARIASEN.rand(nL,(nS-1)*6+5)  SampleTime=AARIAENV.Source_TS
  Random Number2 : RandomNumber  Mean=AARIASEN.aMu  Variance=AARIASEN.aSigma  Seed=AARIASEN.rand(nL,(nS-1)*6+6)  SampleTime=AARIAENV.Source_TS
  Sum1 : Sum  Inputs=|++
  Sum2 : Sum  Inputs=|++
  Sum3 : Sum  Inputs=|++
  Sum4 : Sum  Inputs=++|
  acc in-run bias : simulink/Sources/Ramp  slope=AARIASEN.aBias  start=0  X0=AARIASEN.aInitBias
  acc random walk : UniformRandomNumber  Minimum=-AARIASEN.aWalk  Maximum=AARIASEN.aWalk  Seed=AARIASEN.rand(nL,(nS-1)*6+4)  SampleTime=AARIAENV.Source_TS
  acc random walk1 : UniformRandomNumber  Minimum=-AARIASEN.aWalk  Maximum=AARIASEN.aWalk  Seed=AARIASEN.rand(nL,(nS-1)*6+5)  SampleTime=AARIAENV.Source_TS
  acc random walk2 : UniformRandomNumber  Minimum=-AARIASEN.aWalk  Maximum=AARIASEN.aWalk  Seed=AARIASEN.rand(nL,(nS-1)*6+6)  SampleTime=AARIAENV.Source_TS
  noise : Outport
  wires:
  acc random walk/1 -> Cumulative Sum2/1
  acc in-run bias/1 -> Sum4/1
  Gain2/1 -> noise/1
  Cumulative Sum3/1 -> Sum3/2
  Cumulative Sum2/1 -> Sum1/2
  Sum1/1 -> Mux5/1
  Sum3/1 -> Mux5/3
  Cumulative Sum1/1 -> Sum2/2
  Sum2/1 -> Mux5/2
  acc random walk1/1 -> Cumulative Sum1/1
  acc random walk2/1 -> Cumulative Sum3/1
  Mux5/1 -> Sum4/2
  Sum4/1 -> Gain2/1
  Gain1/1 -> Sum1/1
  Gain5/1 -> Sum2/1
  Gain3/1 -> Sum3/1
  Random Number/1 -> Gain4/1
  Random Number1/1 -> Gain6/1
  Random Number2/1 -> Gain7/1
  Gain4/1 -> Gain1/1
  Gain6/1 -> Gain5/1
  Gain7/1 -> Gain3/1

== system AariaHIABTorqueR2017a2/Joint5/RevoluteMotion/IMU Sensors/Sensor Module2/omega_noise ==
  Cumulative Sum : dspmathops/Cumulative Sum  dim=Channels (running sum)  InputProcessing=Columns as channels (frame based)  reset_popup=None  outputDataTypeStr=Inherit: Same as accumulator  outputLastDataTypeStr=Inherit: Same as accumulator  outputMin=[]  outputMax=[]  roundingMode=Floor  overflowMode=off
      settings: SourceProductName=DSP System Toolbox
  Cumulative Sum1 : dspmathops/Cumulative Sum  dim=Channels (running sum)  InputProcessing=Columns as channels (frame based)  reset_popup=None  outputDataTypeStr=Inherit: Same as accumulator  outputLastDataTypeStr=Inherit: Same as accumulator  outputMin=[]  outputMax=[]  roundingMode=Floor  overflowMode=off
      settings: SourceProductName=DSP System Toolbox
  Cumulative Sum2 : dspmathops/Cumulative Sum  dim=Channels (running sum)  InputProcessing=Columns as channels (frame based)  reset_popup=None  outputDataTypeStr=Inherit: Same as accumulator  outputLastDataTypeStr=Inherit: Same as accumulator  outputMin=[]  outputMax=[]  roundingMode=Floor  overflowMode=off
      settings: SourceProductName=DSP System Toolbox
  Gain1 : Gain  Gain=AARIASEN.ErrorGain
  Gain2 : Gain  Gain=AARIASEN.gNormalGain
  Gain3 : Gain  Gain=AARIASEN.gNormalGain
  Gain4 : Gain  Gain=AARIASEN.gNormalGain
  Mux5 : Mux  Inputs=3
  Random Number : RandomNumber  Mean=AARIASEN.gMu  Variance=AARIASEN.gSigma  Seed=AARIASEN.rand(nL,(nS-1)*6+1)  SampleTime=AARIAENV.Source_TS
  Random Number1 : RandomNumber  Mean=AARIASEN.gMu  Variance=AARIASEN.gSigma  Seed=AARIASEN.rand(nL,(nS-1)*6+2)  SampleTime=AARIAENV.Source_TS
  Random Number2 : RandomNumber  Mean=AARIASEN.gMu  Variance=AARIASEN.gSigma  Seed=AARIASEN.rand(nL,(nS-1)*6+3)  SampleTime=AARIAENV.Source_TS
  Sum1 : Sum  Inputs=|++
  Sum2 : Sum  Inputs=|++
  Sum3 : Sum  Inputs=++|
  Sum4 : Sum  Inputs=|++
  gyro in-run bias : simulink/Sources/Ramp  slope=AARIASEN.gBias  start=0  X0=AARIASEN.gInitBias
  gyro random walk : UniformRandomNumber  Minimum=-AARIASEN.gWalk  Maximum=AARIASEN.gWalk  Seed=AARIASEN.rand(nL,(nS-1)*6+1)  SampleTime=AARIAENV.Source_TS
  gyro random walk1 : UniformRandomNumber  Minimum=-AARIASEN.gWalk  Maximum=AARIASEN.gWalk  Seed=AARIASEN.rand(nL,(nS-1)*6+2)  SampleTime=AARIAENV.Source_TS
  gyro random walk2 : UniformRandomNumber  Minimum=-AARIASEN.gWalk  Maximum=AARIASEN.gWalk  Seed=AARIASEN.rand(nL,(nS-1)*6+3)  SampleTime=AARIAENV.Source_TS
  noise : Outport
  wires:
  gyro in-run bias/1 -> Sum3/1
  Cumulative Sum/1 -> Sum1/2
  gyro random walk/1 -> Cumulative Sum/1
  Gain1/1 -> noise/1
  gyro random walk1/1 -> Cumulative Sum1/1
  gyro random walk2/1 -> Cumulative Sum2/1
  Sum1/1 -> Mux5/1
  Sum2/1 -> Mux5/2
  Cumulative Sum1/1 -> Sum2/2
  Cumulative Sum2/1 -> Sum4/2
  Sum4/1 -> Mux5/3
  Mux5/1 -> Sum3/2
  Sum3/1 -> Gain1/1
  Random Number2/1 -> Gain4/1
  Random Number1/1 -> Gain3/1
  Random Number/1 -> Gain2/1
  Gain2/1 -> Sum1/1
  Gain3/1 -> Sum2/1
  Gain4/1 -> Sum4/1

== system AariaHIABTorqueR2017a2/Base/BaseVSS/BaseEmpty/IMU Base/Sensor Module1/a_noise ==
  Cumulative Sum1 : dspmathops/Cumulative Sum  dim=Channels (running sum)  InputProcessing=Columns as channels (frame based)  reset_popup=None  outputDataTypeStr=Inherit: Same as accumulator  outputLastDataTypeStr=Inherit: Same as accumulator  outputMin=[]  outputMax=[]  roundingMode=Floor  overflowMode=off
      settings: SourceProductName=DSP System Toolbox
  Cumulative Sum2 : dspmathops/Cumulative Sum  dim=Channels (running sum)  InputProcessing=Columns as channels (frame based)  reset_popup=None  outputDataTypeStr=Inherit: Same as accumulator  outputLastDataTypeStr=Inherit: Same as accumulator  outputMin=[]  outputMax=[]  roundingMode=Floor  overflowMode=off
      settings: SourceProductName=DSP System Toolbox
  Cumulative Sum3 : dspmathops/Cumulative Sum  dim=Channels (running sum)  InputProcessing=Columns as channels (frame based)  reset_popup=None  outputDataTypeStr=Inherit: Same as accumulator  outputLastDataTypeStr=Inherit: Same as accumulator  outputMin=[]  outputMax=[]  roundingMode=Floor  overflowMode=off
      settings: SourceProductName=DSP System Toolbox
  Gain1 : Gain  Gain=9.81
  Gain2 : Gain  Gain=AARIASEN.ErrorGain
  Gain3 : Gain  Gain=9.81
  Gain4 : Gain  Gain=AARIASEN.aNormalGain
  Gain5 : Gain  Gain=9.81
  Gain6 : Gain  Gain=AARIASEN.aNormalGain
  Gain7 : Gain  Gain=AARIASEN.aNormalGain
  Mux5 : Mux  Inputs=3
  Random Number : RandomNumber  Mean=AARIASEN.aMu  Variance=AARIASEN.aSigma  Seed=AARIASEN.rand(nL,(nS-1)*6+4)  SampleTime=AARIAENV.Source_TS
  Random Number1 : RandomNumber  Mean=AARIASEN.aMu  Variance=AARIASEN.aSigma  Seed=AARIASEN.rand(nL,(nS-1)*6+5)  SampleTime=AARIAENV.Source_TS
  Random Number2 : RandomNumber  Mean=AARIASEN.aMu  Variance=AARIASEN.aSigma  Seed=AARIASEN.rand(nL,(nS-1)*6+6)  SampleTime=AARIAENV.Source_TS
  Sum1 : Sum  Inputs=|++
  Sum2 : Sum  Inputs=|++
  Sum3 : Sum  Inputs=|++
  Sum4 : Sum  Inputs=++|
  acc in-run bias : simulink/Sources/Ramp  slope=AARIASEN.aBias  start=0  X0=AARIASEN.aInitBias
  acc random walk : UniformRandomNumber  Minimum=-AARIASEN.aWalk  Maximum=AARIASEN.aWalk  Seed=AARIASEN.rand(nL,(nS-1)*6+4)  SampleTime=AARIAENV.Source_TS
  acc random walk1 : UniformRandomNumber  Minimum=-AARIASEN.aWalk  Maximum=AARIASEN.aWalk  Seed=AARIASEN.rand(nL,(nS-1)*6+5)  SampleTime=AARIAENV.Source_TS
  acc random walk2 : UniformRandomNumber  Minimum=-AARIASEN.aWalk  Maximum=AARIASEN.aWalk  Seed=AARIASEN.rand(nL,(nS-1)*6+6)  SampleTime=AARIAENV.Source_TS
  noise : Outport
  wires:
  Gain7/1 -> Gain3/1
  Gain6/1 -> Gain5/1
  Gain4/1 -> Gain1/1
  Random Number2/1 -> Gain7/1
  Random Number1/1 -> Gain6/1
  Random Number/1 -> Gain4/1
  Gain3/1 -> Sum3/1
  Gain5/1 -> Sum2/1
  Gain1/1 -> Sum1/1
  Sum4/1 -> Gain2/1
  Mux5/1 -> Sum4/2
  acc random walk2/1 -> Cumulative Sum3/1
  acc random walk1/1 -> Cumulative Sum1/1
  Sum2/1 -> Mux5/2
  Cumulative Sum1/1 -> Sum2/2
  Sum3/1 -> Mux5/3
  Sum1/1 -> Mux5/1
  Cumulative Sum2/1 -> Sum1/2
  Cumulative Sum3/1 -> Sum3/2
  Gain2/1 -> noise/1
  acc in-run bias/1 -> Sum4/1
  acc random walk/1 -> Cumulative Sum2/1
